simulink model "modello_calcolo_trim_1"  (R2020b)
settings: Solver=ode4  StartTime=0.0  StopTime=0.01  FixedStep=0.01  RelTol=1e-3
values from neighbouring files (symbols this model uses):
  alphavec_rad = deg2rad(alphavec)    [v2021_10_27_calcoloAerodinamica.m]
  b = 2.62    [AENEA2.m]    (also in v2021_10_27_calcoloAerodinamica.m)
  betavec_rad = deg2rad(betavec)    [v2021_10_27_calcoloAerodinamica.m]
  c = .32    (= 0.32)    [AENEA2.m]    (also in calcoloPolari.m = dim(2); v2021_10_27_calcoloAerodinamica.m)
  cbar = .32    (= 0.32)    [v2021_10_27_calcoloAerodinamica.m]
  CD0 = 0.024    [v2021_10_27_calcoloAerodinamica.m]
  CldA = KCldA(1)*180/pi    [AENEA2.m]
  CLdE = KCLdE(1)*180/pi    [AENEA2.m]
  CldR = KCldR(1)*180/pi    [AENEA2.m]
  Clp = -0.4318    [v2021_10_27_calcoloAerodinamica.m]
  CLq = 8.13    [v2021_10_27_calcoloAerodinamica.m]
  Clr = 0.1459    [v2021_10_27_calcoloAerodinamica.m]
  CmdE = KCmdE(1)*180/pi    [AENEA2.m]
  Cmq = -23.24    [v2021_10_27_calcoloAerodinamica.m]
  CndA = KCndA(1)*180/pi    [AENEA2.m]
  CndR = KCndR(1)*180/pi    [AENEA2.m]
  Cnp = 0.007507    [v2021_10_27_calcoloAerodinamica.m]
  Cnr = -0.4872    [v2021_10_27_calcoloAerodinamica.m]
  CYp = 0.050728    [v2021_10_27_calcoloAerodinamica.m]
  CYr = 0.358925    [v2021_10_27_calcoloAerodinamica.m]
  deltaAtrim = 0    [v2021_10_27_avvioSITL.m]
  deltaEtrim = 0    [v2021_10_27_avvioSITL.m]
  deltaRtrim = 0    [v2021_10_27_avvioSITL.m]
  deltaTtrim = 0.1    [v2021_10_27_avvioSITL.m]
  Dprop = 2*Rprop    (= 0.5334)    [v2021_10_27_calcoloAerodinamica.m]
  Jeng = 0    [v2021_10_27_calcoloAerodinamica.m]
  Jprop = mprop*(Dprop^2)/12    (= 0.00422031414)    [v2021_10_27_calcoloAerodinamica.m]
  rACtG = rACtP-rGP    [v2021_10_27_calcoloAerodinamica.m]
  rACwG = rACwP-rGP    [v2021_10_27_calcoloAerodinamica.m]
  rAHRSG = rAHRSP-rGP    [v2021_10_27_calcoloAerodinamica.m]
  rho = P/(287.05*T)    (= 1.16123787958)    [AENEA2.m]    (also in modello_appr_long.m = 1.164; v2021_10_27_calcoloAerodinamica.m = 1.2133)
  rLEG = rLEP-rGP    [v2021_10_27_calcoloAerodinamica.m]
  rmglG = rmglP-rGP    [v2021_10_27_calcoloAerodinamica.m]
  rmgrG = rmgrP-rGP    [v2021_10_27_calcoloAerodinamica.m]
  rngG = rngP-rGP    [v2021_10_27_calcoloAerodinamica.m]
  rNPG = rNPP-rGP    [v2021_10_27_calcoloAerodinamica.m]
  rPG = -rGP    [v2021_10_27_calcoloAerodinamica.m]
  Rprop = 0.2667    [v2021_10_27_calcoloAerodinamica.m]
  S = b*c    (= 0.8384)    [AENEA2.m]    (also in v2021_10_27_calcoloAerodinamica.m)
  W = m*g    [v2021_10_27_calcoloAerodinamica.m]
  Zeng = rPG(3)    [v2021_10_27_calcoloAerodinamica.m]
undefined symbols (not defined in the file or in its folder): CYdA, CYdR, matricepolinomi
libraries: shared6dof x1, aerolibasang x1, simulink x1
settings Model: Creator=Giorgio  LastModifiedBy=39334
settings DataIOCC: ReturnWorkspaceOutputs=off
settings OptimizationCC: BlockReduction=off  OptimizeBlockIOStorage=off  BufferReuse=off  GlobalBufferReuse=off  ExpressionFolding=off  LocalBlockOutputs=off  OptimizeDataStoreBuffers=off  BusAssignmentInplaceUpdate=off
settings DebuggingCC: InitInArrayFormatMsg=none  ArithmeticOperatorsInVariantConditions=warning
settings SFSimCC: CustomCodeUndefinedFunction=UseInterfaceOnly

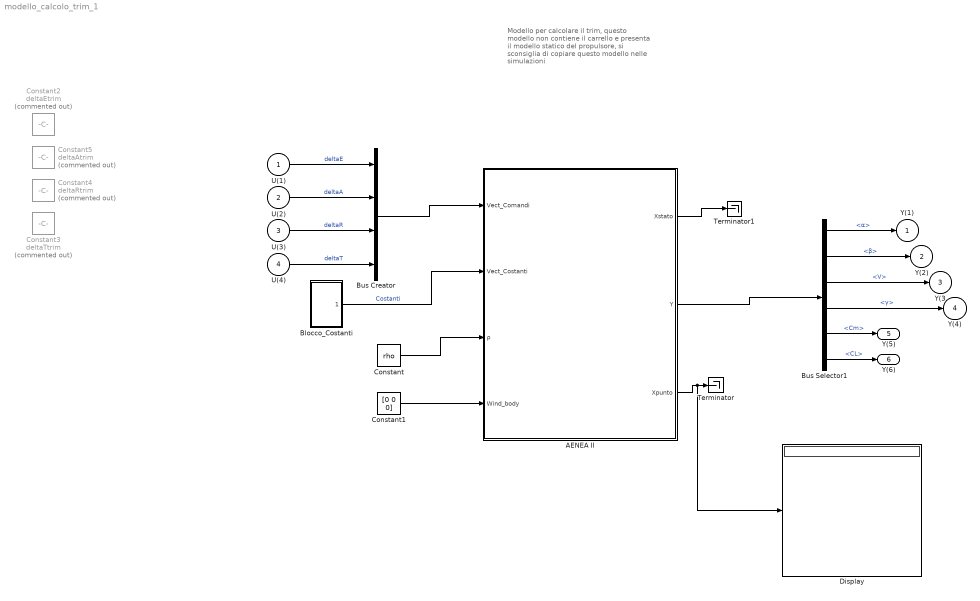
== system modello_calcolo_trim_1 ==
  note: Modello per calcolare il trim, questo modello non contiene il carrello e presenta il modello statico del propulsore, si sconsiglia di copiare questo modello nelle simulazioni
  U(1) : Inport
  U(2) : Inport  Port=2
  U(3) : Inport  Port=3
  U(4) : Inport  Port=4
  "AENEA II " : Subsystem
  Blocco_Costanti : Subsystem
  Bus Creator : BusCreator  Inputs=4
  Bus Selector1 : BusSelector  OutputSignals=Vbpolare.α,Vbpolare.β,Vbpolare.V,γ,Cm,CL
  Constant : Constant  Value=rho
  Constant1 : Constant  Value=[0 0 0]
  Constant2 : Constant  Commented=on  Value=deltaEtrim
  Constant3 : Constant  Commented=on  Value=deltaTtrim
  Constant4 : Constant  Commented=on  Value=deltaRtrim
  Constant5 : Constant  Commented=on  Value=deltaAtrim
  Display : Display
  Terminator : Terminator
  Terminator1 : Terminator
  Y(1) : Outport  VectorParamsAs1DForOutWhenUnconnected=off
  Y(2) : Outport  Port=2  VectorParamsAs1DForOutWhenUnconnected=off
  Y(3 : Outport  Port=3  VectorParamsAs1DForOutWhenUnconnected=off
  Y(4) : Outport  Port=4  VectorParamsAs1DForOutWhenUnconnected=off
  Y(5) : Outport  Port=5  VectorParamsAs1DForOutWhenUnconnected=off
  Y(6) : Outport  Port=6  VectorParamsAs1DForOutWhenUnconnected=off
  wires:
  Blocco_Costanti/1(Vect_Costanti) -> "AENEA II "/2(Vect_Costanti)  "Costanti"
  Constant/1 -> "AENEA II "/3(ρ)
  Bus Creator/1 -> "AENEA II "/1(Vect_Comandi)
  U(2)/1 -> Bus Creator/2  "deltaA"
  U(3)/1 -> Bus Creator/3  "deltaR"
  U(4)/1 -> Bus Creator/4  "deltaT"
  U(1)/1 -> Bus Creator/1  "deltaE"
  "AENEA II "/2(Y) -> Bus Selector1/1
  Bus Selector1/1 -> Y(1)/1  "<α>"
  Bus Selector1/2 -> Y(2)/1  "<β>"
  Bus Selector1/3 -> Y(3/1  "<V>"
  Bus Selector1/4 -> Y(4)/1  "<γ>"
  "AENEA II "/1(Xstato) -> Terminator1/1
  Constant1/1 -> "AENEA II "/4(Wind_body)
  "AENEA II "/3(Xpunto) -> Display/1, Terminator/1
  Bus Selector1/5 -> Y(5)/1  "<Cm>"
  Bus Selector1/6 -> Y(6)/1  "<CL>"

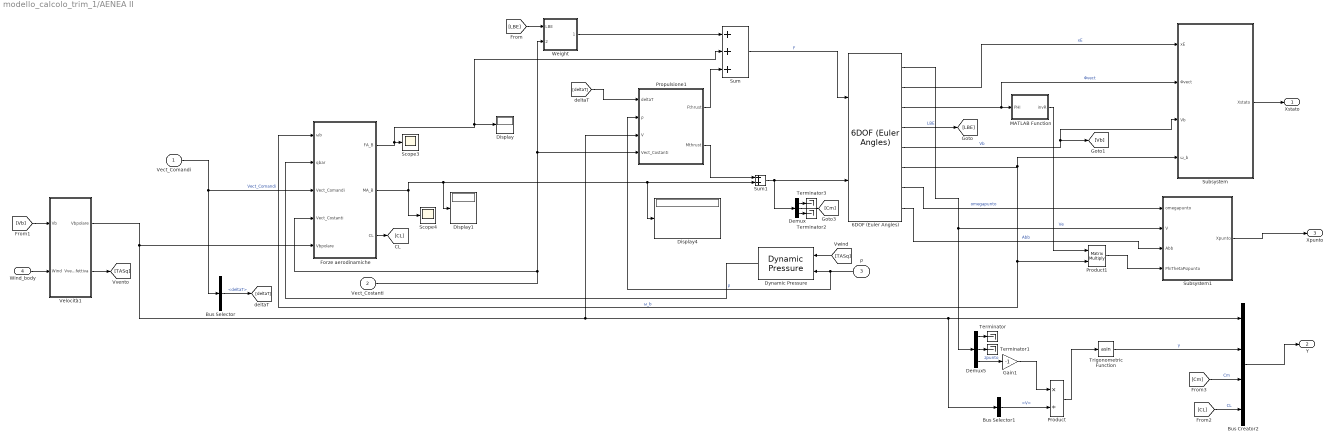
== system modello_calcolo_trim_1/AENEA II  ==
  Vect_Comandi : Inport
  Vect_Costanti : Inport  Port=2
  ρ : Inport  Port=3
  Wind_body : Inport  Port=4
  6DOF (Euler Angles) : shared6dof/6DOF (Euler Angles)  units=Metric (MKS)  mtype=Fixed  rep=Euler Angles  xme_0=State0.Pos0  Vm_0=State0.Vb0  eul_0=State0.PHI0  pm_0=State0.Omega0  mass_0=m  mass_e=0.5  mass_f=2.0  inertia=I  inertia_e=eye(3)  inertia_f=2*eye(3)  k_quat=1.0  vre_flag=on  abi_flag=off  aMode=aMode  xme_statename=''  Vm_statename=''  eul_statename=''  quat_statename=''  pm_statename=''  mass_statename=''
      settings: SourceProductBaseCode=AE,PW,MT,UV,VE,VP
  Bus Creator2 : BusCreator  Inputs=4
  Bus Selector : BusSelector  OutputSignals=deltaT
  Bus Selector1 : BusSelector  OutputSignals=V
  Demux : Demux  Outputs=3
  Demux5 : Demux  Outputs=3
  Display : Display
  Display1 : Display
  Display4 : Display
  Dynamic Pressure : aerolibasang/Dynamic Pressure
  Forze aerodinamiche : Subsystem
  Gain1 : Gain  Gain=-1
  MATLAB Function : MATLAB Function  TreatAsAtomicUnit=on
  Product : Product  Inputs=*/
  Product1 : Product  Multiplication=Matrix(*)
  Propulsione1 : Subsystem
  Scope3 : Scope
  Scope4 : Scope
  Subsystem : Subsystem
  Subsystem1 : Subsystem
  Sum : Sum  Inputs=+++
  Sum1 : Sum  Inputs=2
  Terminator{,1..3} (4 alike) : Terminator
  Trigonometric Function : Trigonometry  Operator=asin
  Velocità1 : Subsystem
  Weight : Subsystem
  Xstato : Outport  VectorParamsAs1DForOutWhenUnconnected=off
  Y : Outport  Port=2  VectorParamsAs1DForOutWhenUnconnected=off
  Xpunto : Outport  Port=3  VectorParamsAs1DForOutWhenUnconnected=off
  wires:
  Sum/1 -> 6DOF (Euler Angles)/1  "F"
  6DOF (Euler Angles)/5 -> Subsystem/3(Vb), [Vb]  "Vb"
  6DOF (Euler Angles)/6 -> Forze aerodinamiche/1(ωb), Product1/2, Subsystem/4(ω_b)  "ω_b"
  6DOF (Euler Angles)/4 -> [LBE]  "LBE"
  Forze aerodinamiche/1(FA_B) -> Sum/2, Display/1, Scope3/1
  Forze aerodinamiche/2(MA_B) -> Display4/1, Sum1/2, Display1/1, Scope4/1
  6DOF (Euler Angles)/1 -> Demux5/1, Subsystem1/2(V)  "Ve"
  Dynamic Pressure/1 -> Forze aerodinamiche/2(qbar)
  Sum1/1 -> 6DOF (Euler Angles)/2, Demux/1
  Weight/1("Forzapeso ") -> Sum/1
  [LBE] -> Weight/1(LBE)
  Vect_Comandi/1 -> Bus Selector/1, Forze aerodinamiche/3(Vect_Comandi)  "Vect_Comandi"
  Bus Selector/1 -> [deltaT]  "<deltaT>"
  Bus Creator2/1 -> Y/1
  Gain1/1 -> Product/1
  Product/1 -> Trigonometric Function/1
  Trigonometric Function/1 -> Bus Creator2/2  "γ"
  ρ/1 -> Propulsione1/2(ρ), Dynamic Pressure/2  "ρ"
  Velocità1/1(Vbpolare) -> Propulsione1/3(V), Bus Selector1/1, Bus Creator2/1, Forze aerodinamiche/5("Vbpolare ")
  [Vb] -> Velocità1/1(Vb)
  6DOF (Euler Angles)/3 -> Subsystem/2(Φvect), MATLAB Function/1(PHI)  "Φvect"
  Bus Selector1/1 -> Product/2  "<V>"
  Wind_body/1 -> Velocità1/2(Wind)
  Forze aerodinamiche/3(CL) -> [CL]
  [Cm] -> Bus Creator2/3  "Cm"
  [CL] -> Bus Creator2/4  "CL"
  6DOF (Euler Angles)/2 -> Subsystem/1(xE)  "xE"
  Subsystem/1("Xstato ") -> Xstato/1
  Demux5/2 -> Terminator1/1
  Demux5/1 -> Terminator/1
  Demux5/3 -> Gain1/1  "zpunto"
  6DOF (Euler Angles)/7 -> Subsystem1/1(omegapunto)  "omegapunto"
  6DOF (Euler Angles)/8 -> Subsystem1/3(Abb)  "Abb"
  Subsystem1/1(Xpunto) -> Xpunto/1
  Product1/1 -> Subsystem1/4("PhiThetaPsipunto ")
  MATLAB Function/1(invR) -> Product1/1
  [deltaT] -> Propulsione1/1("deltaT ")
  Vect_Costanti/1 -> Forze aerodinamiche/4(Vect_Costanti), Weight/2(Vect_Costanti), Propulsione1/4(Vect_Costanti)
  Propulsione1/2(Mthrust) -> Sum1/1
  Propulsione1/1("Fthrust ") -> Sum/3
  Demux/2 -> [Cm]
  Demux/3 -> Terminator2/1
  Demux/1 -> Terminator3/1
  Velocità1/2("Vvento_effettiva ") -> [TASq]
  [TASq] -> Dynamic Pressure/1

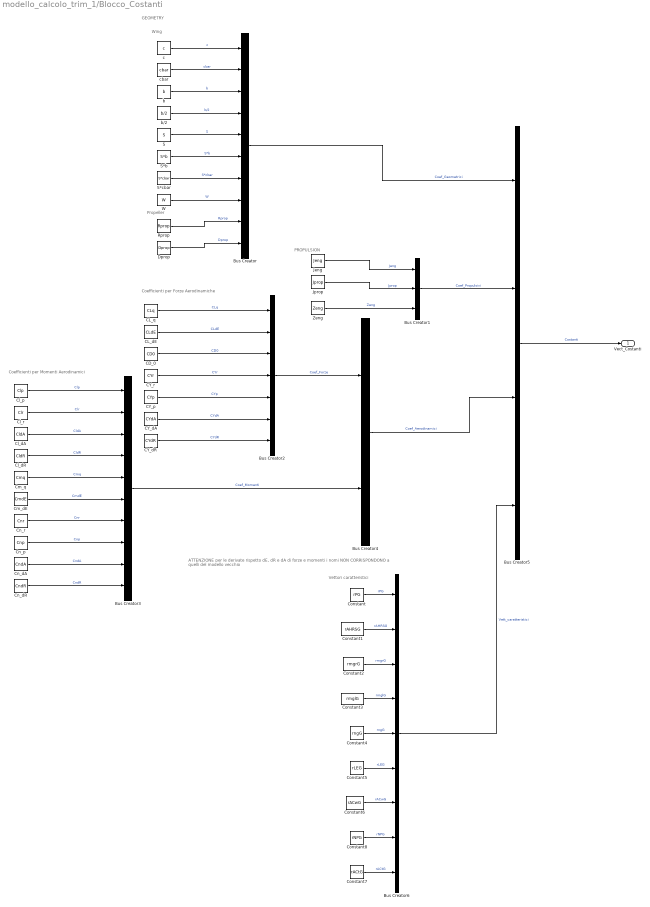
== system modello_calcolo_trim_1/Blocco_Costanti ==
  note: Vettori caratteristici
  note: ATTENZIONE per le derivate rispetto dE, dR e dA di forze e momenti i nomi NON CORRISPONDONO a quelli del modello vecchio
  note: Coefficienti per Forze Aerodinamiche
  note: Coefficienti per Momenti Aerodinamici
  note: Wing
  note: Propeller
  note: PROPULSION
  note: GEOMETRY
  Bus Creator : BusCreator  Inputs=10
  Bus Creator1 : BusCreator  Inputs=3
  Bus Creator2 : BusCreator  Inputs=7
  Bus Creator3 : BusCreator  Inputs=10
  Bus Creator4 : BusCreator  Inputs=2
  Bus Creator5 : BusCreator  Inputs=4
  Bus Creator6 : BusCreator  Inputs=9
  CD_0 : Constant  Value=CD0
  "CL_dE " : Constant  Value=CLdE
  "CL_q " : Constant  Value=CLq
  CY_dA : Constant  Value=CYdA
  CY_dR : Constant  Value=CYdR
  "CY_p " : Constant  Value=CYp
  CY_r : Constant  Value=CYr
  Cl_dA : Constant  Value=CldA
  Cl_dR : Constant  Value=CldR
  "Cl_p " : Constant  Value=Clp
  "Cl_r " : Constant  Value=Clr
  "Cm_dE " : Constant  Value=CmdE
  "Cm_q " : Constant  Value=Cmq
  Cn_dA : Constant  Value=CndA
  "Cn_dR " : Constant  Value=CndR
  "Cn_p " : Constant  Value=Cnp
  "Cn_r " : Constant  Value=Cnr
  Constant : Constant  Value=rPG
  Constant1 : Constant  Value=rAHRSG
  Constant2 : Constant  Value=rmgrG
  Constant3 : Constant  Value=rmglG
  Constant4 : Constant  Value=rngG
  Constant5 : Constant  Value=rLEG
  Constant6 : Constant  Value=rACwG
  Constant7 : Constant  Value=rACtG
  Constant8 : Constant  Value=rNPG
  Dprop : Constant  Value=Dprop
  Jeng : Constant  Value=Jeng
  Jprop : Constant  Value=Jprop
  Rprop : Constant  Value=Rprop
  S : Constant  Value=S
  "S*b " : Constant  Value=S*b
  S*cbar : Constant  Value=S*cbar
  W : Constant  Value=W
  Zeng : Constant  Value=Zeng
  b : Constant  Value=b
  b/2 : Constant  Value=b/2
  c : Constant  Value=c
  "cbar " : Constant  Value=cbar
  Vect_Costanti : Outport  VectorParamsAs1DForOutWhenUnconnected=off
  wires:
  "CY_p "/1 -> Bus Creator2/5  "CYp"
  Cl_dR/1 -> Bus Creator3/4  "CldR"
  "Cn_dR "/1 -> Bus Creator3/10  "CndR"
  "CL_q "/1 -> Bus Creator2/1  "CLq"
  "Cn_p "/1 -> Bus Creator3/8  "Cnp"
  Bus Creator1/1 -> Bus Creator5/2  "Coef_Propulsivi"
  CD_0/1 -> Bus Creator2/3  "CD0"
  Bus Creator4/1 -> Bus Creator5/3  "Coef_Aerodinamici"
  "Cm_dE "/1 -> Bus Creator3/6  "CmdE"
  "Cn_r "/1 -> Bus Creator3/7  "Cnr"
  "Cl_r "/1 -> Bus Creator3/2  "Clr"
  "Cm_q "/1 -> Bus Creator3/5  "Cmq"
  CY_dR/1 -> Bus Creator2/7  "CYdR"
  Cl_dA/1 -> Bus Creator3/3  "CldA"
  CY_dA/1 -> Bus Creator2/6  "CYdA"
  "CL_dE "/1 -> Bus Creator2/2  "CLdE"
  Dprop/1 -> Bus Creator/10  "Dprop"
  Cn_dA/1 -> Bus Creator3/9  "CndA"
  Bus Creator5/1 -> Vect_Costanti/1  "Costanti"
  Bus Creator/1 -> Bus Creator5/1  "Coef_Geometrici"
  Jeng/1 -> Bus Creator1/1  "Jeng"
  c/1 -> Bus Creator/1  "c"
  "S*b "/1 -> Bus Creator/6  "S*b"
  W/1 -> Bus Creator/8  "W"
  Rprop/1 -> Bus Creator/9  "Rprop"
  b/1 -> Bus Creator/3  "b"
  Bus Creator3/1 -> Bus Creator4/2  "Coef_Momenti"
  Bus Creator2/1 -> Bus Creator4/1  "Coef_Forze"
  S*cbar/1 -> Bus Creator/7  "S*cbar"
  Jprop/1 -> Bus Creator1/2  "Jprop"
  b/2/1 -> Bus Creator/4  "b/2"
  "Cl_p "/1 -> Bus Creator3/1  "Clp"
  CY_r/1 -> Bus Creator2/4  "CYr"
  S/1 -> Bus Creator/5  "S"
  "cbar "/1 -> Bus Creator/2  "cbar"
  Zeng/1 -> Bus Creator1/3  "Zeng"
  Constant/1 -> Bus Creator6/1  "rPG"
  Bus Creator6/1 -> Bus Creator5/4  "Vett_caratteristici"
  Constant3/1 -> Bus Creator6/4  "rmglG"
  Constant8/1 -> Bus Creator6/8  "rNPG"
  Constant6/1 -> Bus Creator6/7  "rACwG"
  Constant5/1 -> Bus Creator6/6  "rLEG"
  Constant4/1 -> Bus Creator6/5  "rngG"
  Constant7/1 -> Bus Creator6/9  "rACtG"
  Constant2/1 -> Bus Creator6/3  "rmgrG"
  Constant1/1 -> Bus Creator6/2  "rAHRSG"

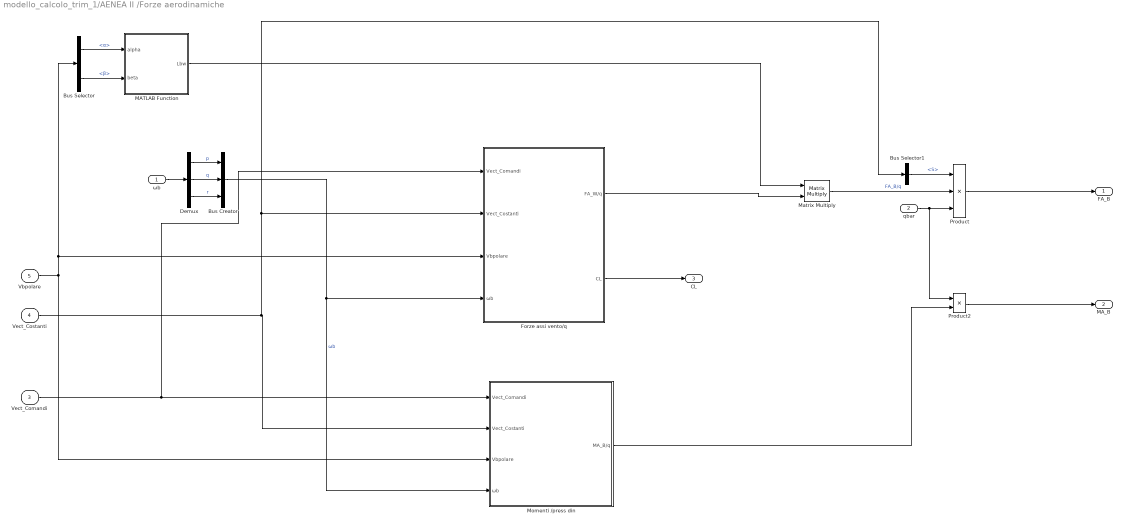
== system modello_calcolo_trim_1/AENEA II /Forze aerodinamiche ==
  ωb : Inport
  qbar : Inport  Port=2
  Vect_Comandi : Inport  Port=3
  Vect_Costanti : Inport  Port=4
  "Vbpolare " : Inport  Port=5
  Bus Creator : BusCreator  Inputs=3
  Bus Selector : BusSelector  OutputSignals=α,β
  Bus Selector1 : BusSelector  OutputSignals=Coef_Geometrici.S
  Demux : Demux  Outputs=3
  Forze assi vento/q : Subsystem
  MATLAB Function : MATLAB Function  TreatAsAtomicUnit=on
  Matrix Multiply : Product  Multiplication=Matrix(*)
  Momenti /press din : Subsystem
  Product : Product  Inputs=3
  Product2 : Product
  FA_B : Outport  VectorParamsAs1DForOutWhenUnconnected=off
  MA_B : Outport  Port=2  VectorParamsAs1DForOutWhenUnconnected=off
  CL : Outport  Port=3  VectorParamsAs1DForOutWhenUnconnected=off
  wires:
  Product2/1 -> MA_B/1
  Product/1 -> FA_B/1
  qbar/1 -> Product/3, Product2/1
  ωb/1 -> Demux/1
  Demux/1 -> Bus Creator/1  "p"
  Demux/2 -> Bus Creator/2  "q"
  Demux/3 -> Bus Creator/3  "r"
  Bus Selector/1 -> MATLAB Function/1(alpha)  "<α>"
  Bus Selector/2 -> MATLAB Function/2(beta)  "<β>"
  MATLAB Function/1(Lbw) -> Matrix Multiply/1
  Matrix Multiply/1 -> Product/2  "FA_B/q"
  Momenti /press din/1(MA_B/q) -> Product2/2
  Forze assi vento/q/1(FA_W/q) -> Matrix Multiply/2
  Vect_Comandi/1 -> Forze assi vento/q/1(Vect_Comandi), Momenti /press din/1(Vect_Comandi)
  "Vbpolare "/1 -> Bus Selector/1, Forze assi vento/q/3("Vbpolare "), Momenti /press din/3("Vbpolare ")
  Bus Creator/1 -> Momenti /press din/4(ωb), Forze assi vento/q/4(ωb)  "ωb"
  Vect_Costanti/1 -> Bus Selector1/1, Forze assi vento/q/2(Vect_Costanti), Momenti /press din/2(Vect_Costanti)
  Bus Selector1/1 -> Product/1  "<S>"
  Forze assi vento/q/2(CL) -> CL/1

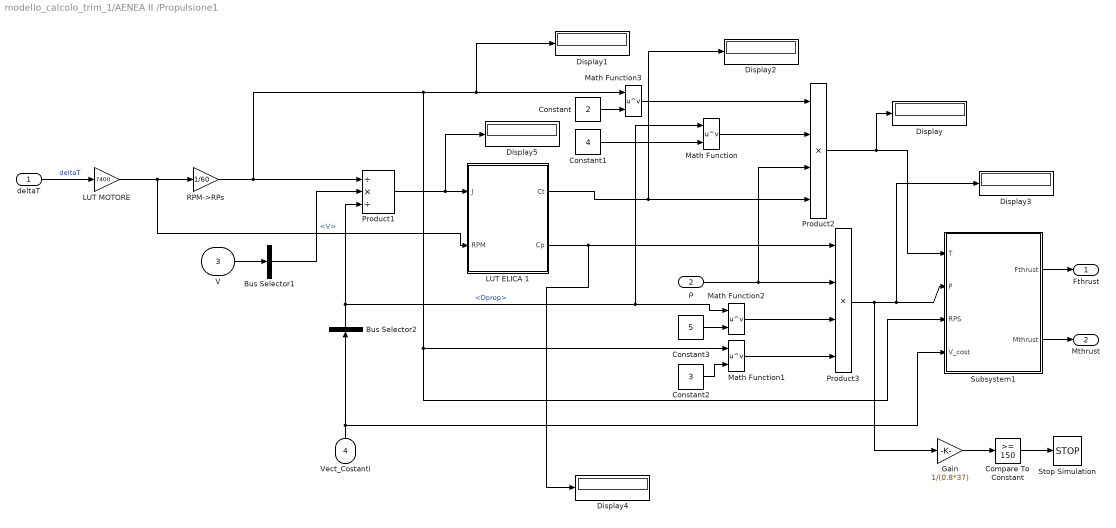
== system modello_calcolo_trim_1/AENEA II /Propulsione1 ==
  "deltaT " : Inport
  ρ : Inport  Port=2
  V : Inport  Port=3
  Vect_Costanti : Inport  Port=4
  Bus Selector1 : BusSelector  OutputSignals=V
  Bus Selector2 : BusSelector  OutputSignals=Coef_Geometrici.Dprop
  Compare To Constant : simulink/Logic and Bit Operations/Compare To Constant  relop=>=  const=150  OutDataTypeStr=boolean
  Constant : Constant  Value=2
  Constant1 : Constant  Value=4
  Constant2 : Constant  Value=3
  Constant3 : Constant  Value=5
  Display{,1..5} (6 alike) : Display
  Gain : Gain  Gain=1/(0.8*37)
  LUT ELICA 1 : Subsystem
  LUT MOTORE : Gain  Gain=7400
  Math Function{,1..3} (4 alike) : Math  Operator=pow  SignedPower=on  SaturateOnIntegerOverflow=on
  Product1 : Product  Inputs=/*/
  Product2 : Product  Inputs=****
  Product3 : Product  Inputs=****
  RPM->RPs : Gain  Gain=1/60
  Stop Simulation : Stop
  Subsystem1 : Subsystem
  "Fthrust " : Outport  VectorParamsAs1DForOutWhenUnconnected=off
  Mthrust : Outport  Port=2  VectorParamsAs1DForOutWhenUnconnected=off
  wires:
  Vect_Costanti/1 -> Subsystem1/4(V_cost), Bus Selector2/1
  "deltaT "/1 -> LUT MOTORE/1  "deltaT"
  LUT MOTORE/1 -> LUT ELICA 1/2(RPM), RPM->RPs/1
  V/1 -> Bus Selector1/1
  Bus Selector1/1 -> Product1/2  "<V>"
  RPM->RPs/1 -> Subsystem1/3(RPS), Math Function1/1, Display1/1, Math Function3/1, Product1/1
  Bus Selector2/1 -> Math Function2/1, Math Function/1, Product1/3  "<Dprop>"
  Product1/1 -> LUT ELICA 1/1(J), Display5/1
  ρ/1 -> Product2/3, Product3/2
  LUT ELICA 1/2(Cp) -> Display4/1, Product3/1
  LUT ELICA 1/1(Ct) -> Display2/1, Product2/4
  Math Function3/1 -> Product2/1
  Math Function/1 -> Product2/2
  Constant/1 -> Math Function3/2
  Constant1/1 -> Math Function/2
  Math Function2/1 -> Product3/3
  Constant3/1 -> Math Function2/2
  Constant2/1 -> Math Function1/2
  Math Function1/1 -> Product3/4
  Product2/1 -> Display/1, Subsystem1/1(T)
  Subsystem1/1(Fthrust) -> "Fthrust "/1
  Subsystem1/2("Mthrust ") -> Mthrust/1
  Product3/1 -> Gain/1, Display3/1, Subsystem1/2(P)
  Gain/1 -> Compare To Constant/1
  Compare To Constant/1 -> Stop Simulation/1

== system modello_calcolo_trim_1/AENEA II /Subsystem ==
  xE : Inport
  Φvect : Inport  Port=2
  Vb : Inport  Port=3
  ω_b : Inport  Port=4
  Bus Creator1 : BusCreator  Inputs=4
  Bus Creator{3..4,8..9} (4 alike) : BusCreator  Inputs=3
  Demux{1..2,6..7} (4 alike) : Demux  Outputs=3
  "Xstato " : Outport  VectorParamsAs1DForOutWhenUnconnected=off
  wires:
  Demux2/3 -> Bus Creator4/3  "r"
  Bus Creator4/1 -> Bus Creator1/3  "ωvect"
  Φvect/1 -> Demux6/1
  Vb/1 -> Demux7/1
  Bus Creator8/1 -> Bus Creator1/2  "PhiThetaPsi"
  Demux1/3 -> Bus Creator3/3  "h"
  Demux2/2 -> Bus Creator4/2  "q"
  Demux2/1 -> Bus Creator4/1  "p"
  Bus Creator3/1 -> Bus Creator1/4  "xyz"
  ω_b/1 -> Demux2/1
  Demux6/3 -> Bus Creator8/3  "Psi"
  Demux6/1 -> Bus Creator8/1  "Phi"
  Demux1/1 -> Bus Creator3/1  "x"
  Demux7/1 -> Bus Creator9/1  "u"
  Demux7/3 -> Bus Creator9/3  "w"
  Bus Creator9/1 -> Bus Creator1/1  "uvw"
  Demux1/2 -> Bus Creator3/2  "y"
  Demux7/2 -> Bus Creator9/2  "v"
  Demux6/2 -> Bus Creator8/2  "Theta"
  Bus Creator1/1 -> "Xstato "/1  "Xstato"
  xE/1 -> Demux1/1

== system modello_calcolo_trim_1/AENEA II /Subsystem1 ==
  omegapunto : Inport
  V : Inport  Port=2
  Abb : Inport  Port=3
  "PhiThetaPsipunto " : Inport  Port=4
  Bus Creator{5,7,10..11} (4 alike) : BusCreator  Inputs=3
  Bus Creator6 : BusCreator  Inputs=4
  Demux{3..4,8..9} (4 alike) : Demux  Outputs=3
  Xpunto : Outport  VectorParamsAs1DForOutWhenUnconnected=off
  wires:
  Demux4/3 -> Bus Creator7/3  "wpunto"
  Demux3/1 -> Bus Creator5/1  "ppunto"
  Demux4/2 -> Bus Creator7/2  "vpunto"
  Demux8/2 -> Bus Creator10/2  "Thetapunto"
  Bus Creator10/1 -> Bus Creator6/2  "EulerAnglespunto"
  Demux3/2 -> Bus Creator5/2  "qpunto"
  Demux4/1 -> Bus Creator7/1  "upunto"
  V/1 -> Demux9/1
  Demux8/1 -> Bus Creator10/1  "Phipunto"
  Bus Creator11/1 -> Bus Creator6/4  "xyzpunto"
  Demux8/3 -> Bus Creator10/3  "Psipunto"
  Demux3/3 -> Bus Creator5/3  "rpunto"
  Demux9/2 -> Bus Creator11/2  "Yepunto"
  Bus Creator7/1 -> Bus Creator6/1  "Vbpunto"
  Bus Creator5/1 -> Bus Creator6/3  "ωpunto"
  Demux9/1 -> Bus Creator11/1  "Xepunto"
  Demux9/3 -> Bus Creator11/3  "Zepunto"
  "PhiThetaPsipunto "/1 -> Demux8/1
  omegapunto/1 -> Demux3/1
  Abb/1 -> Demux4/1
  Bus Creator6/1 -> Xpunto/1

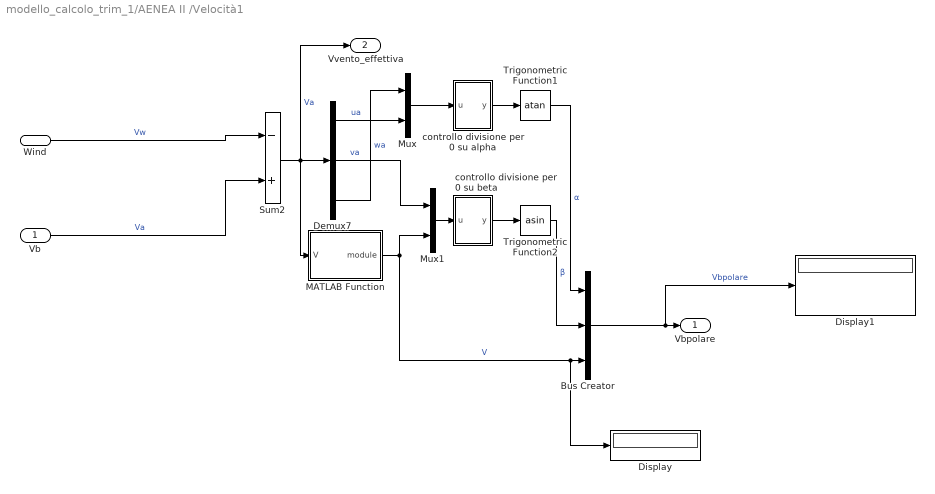
== system modello_calcolo_trim_1/AENEA II /Velocità1 ==
  Vb : Inport
  Wind : Inport  Port=2
  Bus Creator : BusCreator  Inputs=3
  Demux7 : Demux  Outputs=3
  Display : Display
  Display1 : Display
  MATLAB Function : MATLAB Function  TreatAsAtomicUnit=on
  Mux : Mux  Inputs=2
  Mux1 : Mux  Inputs=2
  Sum2 : Sum  Inputs=-+
  Trigonometric Function1 : Trigonometry  Operator=atan
  Trigonometric Function2 : Trigonometry  Operator=asin
  controllo divisione per 0 su alpha : MATLAB Function  TreatAsAtomicUnit=on
  controllo divisione per 0 su beta : MATLAB Function  TreatAsAtomicUnit=on
  Vbpolare : Outport  VectorParamsAs1DForOutWhenUnconnected=off
  "Vvento_effettiva " : Outport  Port=2  VectorParamsAs1DForOutWhenUnconnected=off
  wires:
  Bus Creator/1 -> Display1/1, Vbpolare/1  "Vbpolare"
  Trigonometric Function1/1 -> Bus Creator/1  "α"
  MATLAB Function/1(module) -> Mux1/2, Display/1, Bus Creator/3  "V"
  controllo divisione per 0 su alpha/1(y) -> Trigonometric Function1/1
  controllo divisione per 0 su beta/1(y) -> Trigonometric Function2/1
  Trigonometric Function2/1 -> Bus Creator/2  "β"
  Vb/1 -> Sum2/2  "Va"
  Sum2/1 -> "Vvento_effettiva "/1, MATLAB Function/1(V), Demux7/1  "Va"
  Mux/1 -> controllo divisione per 0 su alpha/1(u)
  Demux7/3 -> Mux/1  "wa"
  Demux7/1 -> Mux/2  "ua"
  Mux1/1 -> controllo divisione per 0 su beta/1(u)
  Demux7/2 -> Mux1/1  "va"
  Wind/1 -> Sum2/1  "Vw"

== system modello_calcolo_trim_1/AENEA II /Weight ==
  LBE : Inport
  Vect_Costanti : Inport  Port=2
  Bus Selector : BusSelector  OutputSignals=Coef_Geometrici.W
  Display3 : Display
  Product3 : Product  Multiplication=Matrix(*)
  "Forzapeso " : Outport  VectorParamsAs1DForOutWhenUnconnected=off
  wires:
  Product3/1 -> "Forzapeso "/1, Display3/1
  LBE/1 -> Product3/1
  Vect_Costanti/1 -> Bus Selector/1
  Bus Selector/1 -> Product3/2  "<W>"

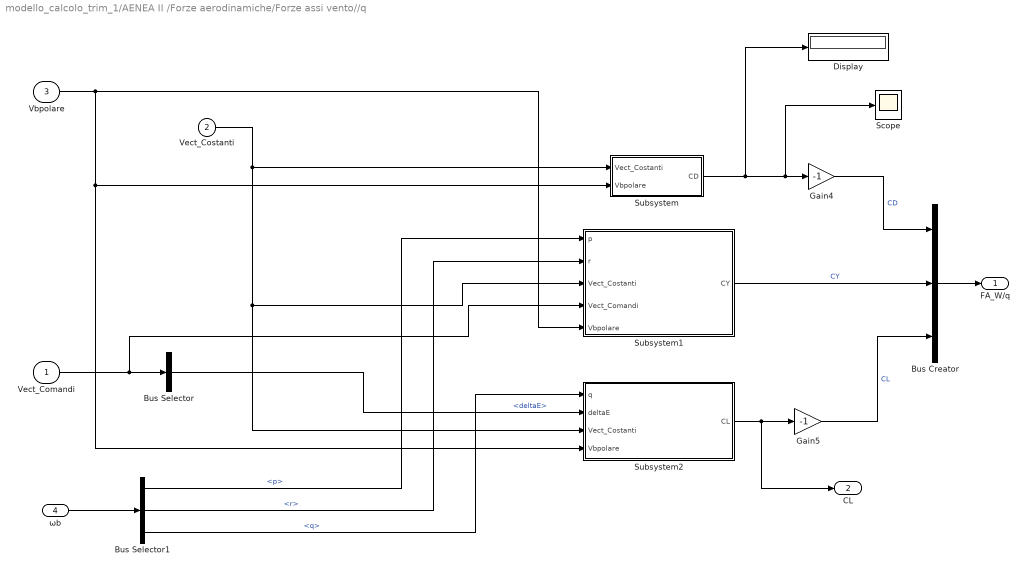
== system modello_calcolo_trim_1/AENEA II /Forze aerodinamiche/Forze assi vento//q ==
  Vect_Comandi : Inport
  Vect_Costanti : Inport  Port=2
  "Vbpolare " : Inport  Port=3
  ωb : Inport  Port=4
  Bus Creator : BusCreator  Inputs=3
  Bus Selector : BusSelector  OutputSignals=deltaE
  Bus Selector1 : BusSelector  OutputSignals=p,r,q
  Display : Display
  Gain4 : Gain  Gain=-1
  Gain5 : Gain  Gain=-1
  Scope : Scope
  Subsystem : Subsystem
  Subsystem1 : Subsystem
  Subsystem2 : Subsystem
  FA_W/q : Outport  VectorParamsAs1DForOutWhenUnconnected=off
  CL : Outport  Port=2  VectorParamsAs1DForOutWhenUnconnected=off
  wires:
  Bus Selector/1 -> Subsystem2/2(deltaE)  "<deltaE>"
  Subsystem/1(CD) -> Display/1, Scope/1, Gain4/1
  Subsystem2/1(CL) -> CL/1, Gain5/1
  Vect_Costanti/1 -> Subsystem2/3(Vect_Costanti), Subsystem1/3(Vect_Costanti), Subsystem/1(Vect_Costanti)
  Vect_Comandi/1 -> Subsystem1/4(Vect_Comandi), Bus Selector/1
  "Vbpolare "/1 -> Subsystem1/5("Vbpolare "), Subsystem2/4("Vbpolare "), Subsystem/2("Vbpolare ")
  ωb/1 -> Bus Selector1/1
  Bus Selector1/1 -> Subsystem1/1(p)  "<p>"
  Bus Selector1/3 -> Subsystem2/1(q)  "<q>"
  Bus Selector1/2 -> Subsystem1/2(r)  "<r>"
  Bus Creator/1 -> FA_W/q/1
  Gain5/1 -> Bus Creator/3  "CL"
  Subsystem1/1("CY ") -> Bus Creator/2  "CY"
  Gain4/1 -> Bus Creator/1  "CD"

== system modello_calcolo_trim_1/AENEA II /Forze aerodinamiche/Momenti //press din ==
  Vect_Comandi : Inport
  Vect_Costanti : Inport  Port=2
  "Vbpolare " : Inport  Port=3
  ωb : Inport  Port=4
  Bus Creator : BusCreator  Inputs=3
  Bus Selector : BusSelector  OutputSignals=Coef_Geometrici.S*b,Coef_Geometrici.S*cbar
  Product : Product
  Product1 : Product
  Product3 : Product
  Subsystem3 : Subsystem
  Subsystem4 : Subsystem
  Subsystem5 : Subsystem
  MA_B/q : Outport  VectorParamsAs1DForOutWhenUnconnected=off
  wires:
  Subsystem5/1(Cn) -> Product3/2
  Subsystem4/1(Cm) -> Product1/2
  Subsystem3/1(Cl) -> Product/2
  Vect_Costanti/1 -> Bus Selector/1, Subsystem3/1(Vect_Costanti), Subsystem5/1(Vect_Costanti), Subsystem4/1(Vect_Costanti)
  Vect_Comandi/1 -> Subsystem4/2(Vect_Comandi), Subsystem3/2(Vect_Comandi), Subsystem5/2(Vect_Comandi)
  "Vbpolare "/1 -> Subsystem5/3("Vbpolare "), Subsystem4/3("Vbpolare "), Subsystem3/3("Vbpolare ")
  ωb/1 -> Subsystem5/4(ωb), Subsystem4/4(ωb), Subsystem3/4(ωb)
  Bus Selector/1 -> Product3/1, Product/1  "<S*b>"
  Bus Selector/2 -> Product1/1  "<S*cbar>"
  Bus Creator/1 -> MA_B/q/1
  Product/1 -> Bus Creator/1  "Cl"
  Product1/1 -> Bus Creator/2  "Cm"
  Product3/1 -> Bus Creator/3  "Cn"

== system modello_calcolo_trim_1/AENEA II /Propulsione1/LUT ELICA 1 ==
  J : Inport
  RPM : Inport  Port=2
  Constant : Constant  Value=matricepolinomi  VectorParams1D=off
  MATLAB Function : MATLAB Function  TreatAsAtomicUnit=on
  Ct : Outport  VectorParamsAs1DForOutWhenUnconnected=off
  Cp : Outport  Port=2  VectorParamsAs1DForOutWhenUnconnected=off
  wires:
  MATLAB Function/2(Cp) -> Cp/1  "Cp"
  J/1 -> MATLAB Function/1(J)
  Constant/1 -> MATLAB Function/3(matricepolinomi)
  MATLAB Function/1(Ct) -> Ct/1  "Ct"
  RPM/1 -> MATLAB Function/2(RPM)

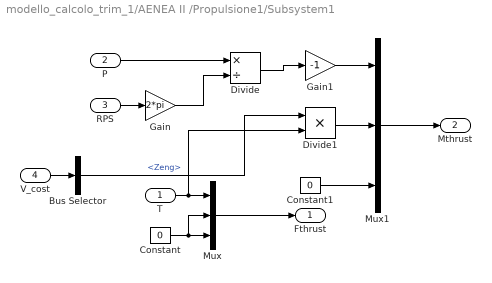
== system modello_calcolo_trim_1/AENEA II /Propulsione1/Subsystem1 ==
  T : Inport
  P : Inport  Port=2
  RPS : Inport  Port=3
  V_cost : Inport  Port=4
  Bus Selector : BusSelector  OutputSignals=Coef_Propulsivi.Zeng
  Constant : Constant  Value=0
  Constant1 : Constant  Value=0
  Divide : Product  Inputs=*/
  Divide1 : Product  Inputs=**
  Gain : Gain  Gain=2*pi
  Gain1 : Gain  Gain=-1
  Mux : Mux  Inputs=3
  Mux1 : Mux  Inputs=3
  Fthrust : Outport  VectorParamsAs1DForOutWhenUnconnected=off
  "Mthrust " : Outport  Port=2  VectorParamsAs1DForOutWhenUnconnected=off
  wires:
  T/1 -> Divide1/2, Mux/1
  Constant/1 -> Mux/2, Mux/3
  Mux/1 -> Fthrust/1
  RPS/1 -> Gain/1
  P/1 -> Divide/1
  Gain/1 -> Divide/2
  Gain1/1 -> Mux1/1
  Divide/1 -> Gain1/1
  Divide1/1 -> Mux1/2
  Constant1/1 -> Mux1/3
  Mux1/1 -> "Mthrust "/1
  V_cost/1 -> Bus Selector/1
  Bus Selector/1 -> Divide1/1  "<Zeng>"

== system modello_calcolo_trim_1/AENEA II /Forze aerodinamiche/Forze assi vento//q/Subsystem ==
  note: CD=CD(alpha_x,beta)
  Vect_Costanti : Inport
  "Vbpolare " : Inport  Port=2
  2-D Lookup Table : Lookup_n-D  BreakpointsForDimension1=alphavec_rad  BreakpointsForDimension2=betavec_rad  Table=CD(2:end,2:end)  InternalRulePriority=Speed  RndMeth=Simplest  InputSameDT=on
      settings: InputPortMap=u0,u1
  Bus Selector : BusSelector  OutputSignals=Coef_Aerodinamici.Coef_Forze.CD0
  Bus Selector1 : BusSelector  OutputSignals=α,β
  Sum1 : Sum  Inputs=|++
  CD : Outport  VectorParamsAs1DForOutWhenUnconnected=off
  wires:
  2-D Lookup Table/1 -> Sum1/1
  Sum1/1 -> CD/1
  Bus Selector/1 -> Sum1/2  "<CD0>"
  Vect_Costanti/1 -> Bus Selector/1
  Bus Selector1/1 -> 2-D Lookup Table/1  "<α>"
  "Vbpolare "/1 -> Bus Selector1/1
  Bus Selector1/2 -> 2-D Lookup Table/2  "<β>"

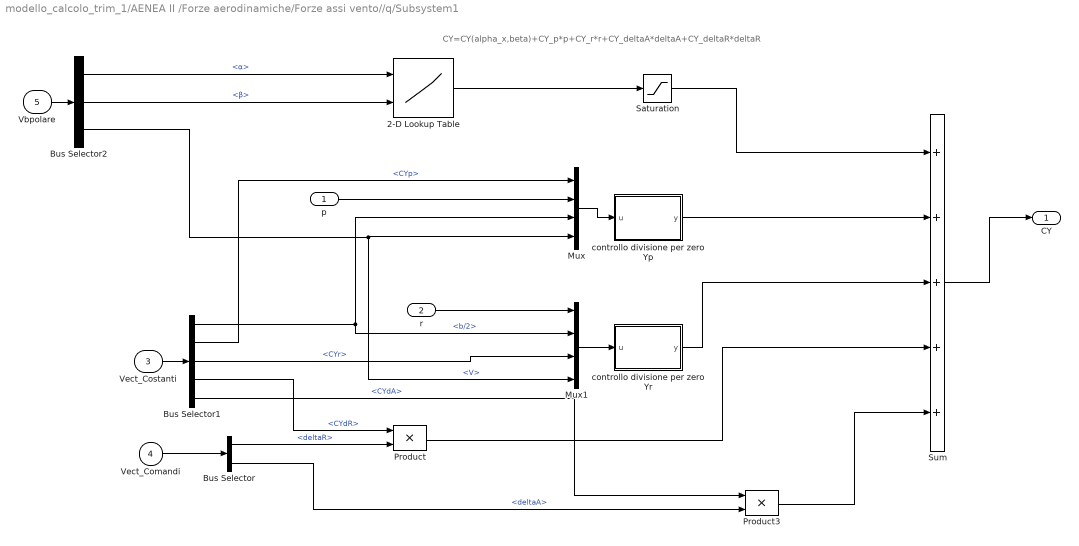
== system modello_calcolo_trim_1/AENEA II /Forze aerodinamiche/Forze assi vento//q/Subsystem1 ==
  note: CY=CY(alpha_x,beta)+CY_p*p+CY_r*r+CY_deltaA*deltaA+CY_deltaR*deltaR
  p : Inport
  r : Inport  Port=2
  Vect_Costanti : Inport  Port=3
  Vect_Comandi : Inport  Port=4
  "Vbpolare " : Inport  Port=5
  2-D Lookup Table : Lookup_n-D  BreakpointsForDimension1=alphavec_rad  BreakpointsForDimension2=betavec_rad  Table=CY(2:end,2:end)  InternalRulePriority=Speed  RndMeth=Simplest  InputSameDT=on
      settings: InputPortMap=u0,u1
  Bus Selector : BusSelector  OutputSignals=deltaR,deltaA
  Bus Selector1 : BusSelector  OutputSignals=Coef_Geometrici.b/2,Coef_Aerodinamici.Coef_Forze.CYp,Coef_Aerodinamici.Coef_Forze.CYr,Coef_Aerodinamici.Coef_Forze.CYdR,Coef_Aerodinamici.Coef_Forze.CYdA
  Bus Selector2 : BusSelector  OutputSignals=α,β,V
  Mux : Mux
  Mux1 : Mux
  Product : Product
  Product3 : Product
  Saturation : Saturate  UpperLimit=0.1  LowerLimit=-0.1
  Sum : Sum  Inputs=5
  "controllo divisione per zero Yp " : MATLAB Function  TreatAsAtomicUnit=on
  controllo divisione per zero Yr : MATLAB Function  TreatAsAtomicUnit=on
  "CY " : Outport  VectorParamsAs1DForOutWhenUnconnected=off
  wires:
  Bus Selector1/2 -> Mux/1  "<CYp>"
  p/1 -> Mux/2
  "controllo divisione per zero Yp "/1(y) -> Sum/2
  Sum/1 -> "CY "/1
  r/1 -> Mux1/1
  2-D Lookup Table/1 -> Saturation/1
  Bus Selector1/4 -> Product/1  "<CYdR>"
  Bus Selector/1 -> Product/2  "<deltaR>"
  Bus Selector1/5 -> Product3/1  "<CYdA>"
  Bus Selector/2 -> Product3/2  "<deltaA>"
  Product/1 -> Sum/4
  Product3/1 -> Sum/5
  Vect_Comandi/1 -> Bus Selector/1
  Vect_Costanti/1 -> Bus Selector1/1
  Bus Selector1/3 -> Mux1/3  "<CYr>"
  Bus Selector1/1 -> Mux/3, Mux1/2  "<b/2>"
  Bus Selector2/1 -> 2-D Lookup Table/1  "<α>"
  "Vbpolare "/1 -> Bus Selector2/1
  Bus Selector2/3 -> Mux/4, Mux1/4  "<V>"
  Bus Selector2/2 -> 2-D Lookup Table/2  "<β>"
  Mux/1 -> "controllo divisione per zero Yp "/1(u)
  Mux1/1 -> controllo divisione per zero Yr/1(u)
  controllo divisione per zero Yr/1(y) -> Sum/3
  Saturation/1 -> Sum/1

== system modello_calcolo_trim_1/AENEA II /Forze aerodinamiche/Forze assi vento//q/Subsystem2 ==
  note: CL=CL(ALPHA_X,BETA)+CL_q*q+CL_de*de
  q : Inport
  deltaE : Inport  Port=2
  Vect_Costanti : Inport  Port=3
  "Vbpolare " : Inport  Port=4
  2-D Lookup Table : Lookup_n-D  BreakpointsForDimension1=alphavec_rad  BreakpointsForDimension2=betavec_rad  Table=CL(2:end,2:end)  InternalRulePriority=Speed  RndMeth=Simplest  InputSameDT=on
      settings: InputPortMap=u0,u1
  Bus Selector : BusSelector  OutputSignals=Coef_Aerodinamici.Coef_Forze.CLq,Coef_Aerodinamici.Coef_Forze.CLdE,Coef_Geometrici.cbar
  Bus Selector1 : BusSelector  OutputSignals=α,β,V
  Gain1 : Gain  Gain=2
  Mux : Mux
  Product4 : Product
  Sum : Sum  Inputs=3
  "controllo divisione per zero Lq " : MATLAB Function  TreatAsAtomicUnit=on
  CL : Outport  VectorParamsAs1DForOutWhenUnconnected=off
  wires:
  Sum/1 -> CL/1
  q/1 -> Mux/2
  Bus Selector/1 -> Mux/1  "<CLq>"
  Bus Selector/2 -> Product4/1  "<CLdE>"
  deltaE/1 -> Product4/2
  "controllo divisione per zero Lq "/1(y) -> Sum/2
  Product4/1 -> Sum/3
  2-D Lookup Table/1 -> Sum/1
  Vect_Costanti/1 -> Bus Selector/1
  Gain1/1 -> Mux/4
  Bus Selector/3 -> Mux/3  "<cbar>"
  Bus Selector1/1 -> 2-D Lookup Table/1  "<α>"
  "Vbpolare "/1 -> Bus Selector1/1
  Bus Selector1/3 -> Gain1/1  "<V>"
  Bus Selector1/2 -> 2-D Lookup Table/2  "<β>"
  Mux/1 -> "controllo divisione per zero Lq "/1(u)

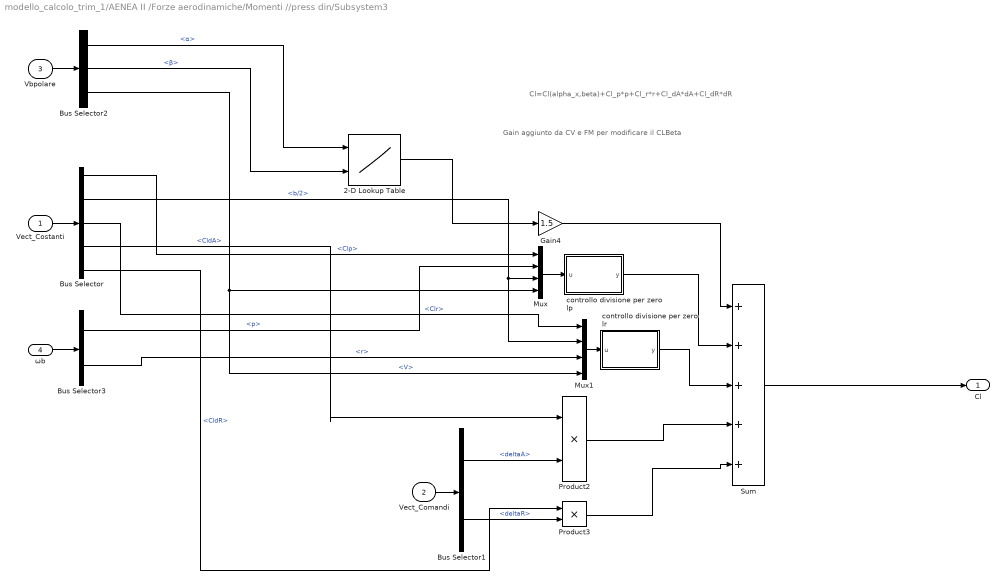
== system modello_calcolo_trim_1/AENEA II /Forze aerodinamiche/Momenti //press din/Subsystem3 ==
  note: Gain aggiunto da CV e FM per modificare il CLBeta
  note: Cl=Cl(alpha_x,beta)+Cl_p*p+Cl_r*r+Cl_dA*dA+Cl_dR*dR
  Vect_Costanti : Inport
  Vect_Comandi : Inport  Port=2
  "Vbpolare " : Inport  Port=3
  ωb : Inport  Port=4
  2-D Lookup Table : Lookup_n-D  BreakpointsForDimension1=alphavec_rad  BreakpointsForDimension2=betavec_rad  Table=Cl(2:end,2:end)  InternalRulePriority=Speed  RndMeth=Simplest  InputSameDT=on
      settings: InputPortMap=u0,u1
  Bus Selector : BusSelector  OutputSignals=Coef_Aerodinamici.Coef_Momenti.Clp,Coef_Geometrici.b/2,Coef_Aerodinamici.Coef_Momenti.Clr,Coef_Aerodinamici.Coef_Momenti.CldA,Coef_Aerodinamici.Coef_Momenti.CldR
  Bus Selector1 : BusSelector  OutputSignals=deltaA,deltaR
  Bus Selector2 : BusSelector  OutputSignals=α,β,V
  Bus Selector3 : BusSelector  OutputSignals=p,r
  Gain4 : Gain  Gain=1.5
  Mux : Mux
  Mux1 : Mux
  Product2 : Product
  Product3 : Product
  Sum : Sum  Inputs=5
  "controllo divisione per zero lp " : MATLAB Function  TreatAsAtomicUnit=on
  "controllo divisione per zero lr " : MATLAB Function  TreatAsAtomicUnit=on
  Cl : Outport  VectorParamsAs1DForOutWhenUnconnected=off
  wires:
  Sum/1 -> Cl/1
  Bus Selector/3 -> Mux1/1  "<Clr>"
  Bus Selector1/2 -> Product3/2  "<deltaR>"
  Bus Selector1/1 -> Product2/2  "<deltaA>"
  Product3/1 -> Sum/5
  Product2/1 -> Sum/4
  "controllo divisione per zero lp "/1(y) -> Sum/2
  2-D Lookup Table/1 -> Gain4/1
  Gain4/1 -> Sum/1
  Vect_Costanti/1 -> Bus Selector/1
  Bus Selector/1 -> Mux/1  "<Clp>"
  Bus Selector/5 -> Product3/1  "<CldR>"
  Bus Selector/4 -> Product2/1  "<CldA>"
  Bus Selector/2 -> Mux1/2, Mux/3  "<b/2>"
  Vect_Comandi/1 -> Bus Selector1/1
  Bus Selector2/1 -> 2-D Lookup Table/1  "<α>"
  "Vbpolare "/1 -> Bus Selector2/1
  Bus Selector2/3 -> Mux1/4, Mux/4  "<V>"
  Bus Selector2/2 -> 2-D Lookup Table/2  "<β>"
  ωb/1 -> Bus Selector3/1
  Bus Selector3/1 -> Mux/2  "<p>"
  Bus Selector3/2 -> Mux1/3  "<r>"
  Mux/1 -> "controllo divisione per zero lp "/1(u)
  Mux1/1 -> "controllo divisione per zero lr "/1(u)
  "controllo divisione per zero lr "/1(y) -> Sum/3

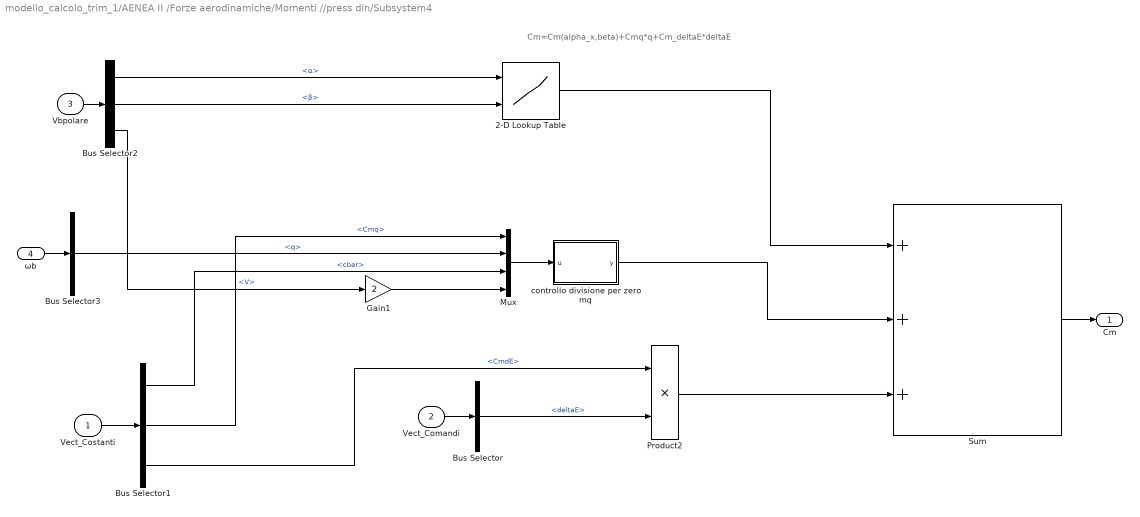
== system modello_calcolo_trim_1/AENEA II /Forze aerodinamiche/Momenti //press din/Subsystem4 ==
  note: Cm=Cm(alpha_x,beta)+Cmq*q+Cm_deltaE*deltaE
  Vect_Costanti : Inport
  Vect_Comandi : Inport  Port=2
  "Vbpolare " : Inport  Port=3
  ωb : Inport  Port=4
  2-D Lookup Table : Lookup_n-D  BreakpointsForDimension1=alphavec_rad  BreakpointsForDimension2=betavec_rad  Table=Cm(2:end,2:end)  InternalRulePriority=Speed  RndMeth=Simplest  InputSameDT=on
      settings: InputPortMap=u0,u1
  Bus Selector : BusSelector  OutputSignals=deltaE
  Bus Selector1 : BusSelector  OutputSignals=Coef_Geometrici.cbar,Coef_Aerodinamici.Coef_Momenti.Cmq,Coef_Aerodinamici.Coef_Momenti.CmdE
  Bus Selector2 : BusSelector  OutputSignals=α,β,V
  Bus Selector3 : BusSelector  OutputSignals=q
  Gain1 : Gain  Gain=2
  Mux : Mux
  Product2 : Product
  Sum : Sum  Inputs=3
  "controllo divisione per zero mq " : MATLAB Function  TreatAsAtomicUnit=on
  Cm : Outport  VectorParamsAs1DForOutWhenUnconnected=off
  wires:
  Bus Selector1/2 -> Mux/1  "<Cmq>"
  Sum/1 -> Cm/1
  Gain1/1 -> Mux/4
  Bus Selector1/3 -> Product2/1  "<CmdE>"
  Bus Selector/1 -> Product2/2  "<deltaE>"
  Product2/1 -> Sum/3
  2-D Lookup Table/1 -> Sum/1
  Vect_Comandi/1 -> Bus Selector/1
  Vect_Costanti/1 -> Bus Selector1/1
  Bus Selector1/1 -> Mux/3  "<cbar>"
  Bus Selector2/3 -> Gain1/1  "<V>"
  "Vbpolare "/1 -> Bus Selector2/1
  Bus Selector2/1 -> 2-D Lookup Table/1  "<α>"
  Bus Selector2/2 -> 2-D Lookup Table/2  "<β>"
  ωb/1 -> Bus Selector3/1
  Bus Selector3/1 -> Mux/2  "<q>"
  Mux/1 -> "controllo divisione per zero mq "/1(u)
  "controllo divisione per zero mq "/1(y) -> Sum/2

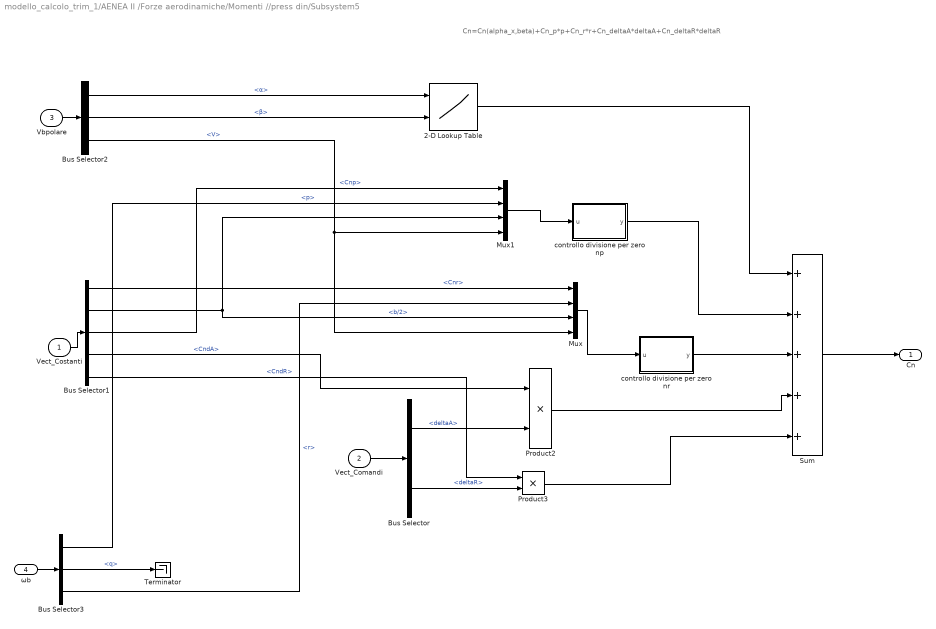
== system modello_calcolo_trim_1/AENEA II /Forze aerodinamiche/Momenti //press din/Subsystem5 ==
  note: Cn=Cn(alpha_x,beta)+Cn_p*p+Cn_r*r+Cn_deltaA*deltaA+Cn_deltaR*deltaR
  Vect_Costanti : Inport
  Vect_Comandi : Inport  Port=2
  "Vbpolare " : Inport  Port=3
  ωb : Inport  Port=4
  2-D Lookup Table : Lookup_n-D  BreakpointsForDimension1=alphavec_rad  BreakpointsForDimension2=betavec_rad  Table=Cn(2:end,2:end)  InternalRulePriority=Speed  RndMeth=Simplest  InputSameDT=on
      settings: InputPortMap=u0,u1
  Bus Selector : BusSelector  OutputSignals=deltaA,deltaR
  Bus Selector1 : BusSelector  OutputSignals=Coef_Aerodinamici.Coef_Momenti.Cnr,Coef_Geometrici.b/2,Coef_Aerodinamici.Coef_Momenti.Cnp,Coef_Aerodinamici.Coef_Momenti.CndA,Coef_Aerodinamici.Coef_Momenti.CndR
  Bus Selector2 : BusSelector  OutputSignals=α,β,V
  Bus Selector3 : BusSelector  OutputSignals=p,q,r
  Mux : Mux
  Mux1 : Mux
  Product2 : Product
  Product3 : Product
  Sum : Sum  Inputs=5
  Terminator : Terminator
  "controllo divisione per zero np " : MATLAB Function  TreatAsAtomicUnit=on
  "controllo divisione per zero nr " : MATLAB Function  TreatAsAtomicUnit=on
  Cn : Outport  VectorParamsAs1DForOutWhenUnconnected=off
  wires:
  Bus Selector1/3 -> Mux1/1  "<Cnp>"
  Product2/1 -> Sum/4
  Product3/1 -> Sum/5
  Sum/1 -> Cn/1
  Bus Selector1/1 -> Mux/1  "<Cnr>"
  Bus Selector1/5 -> Product3/1  "<CndR>"
  Bus Selector/2 -> Product3/2  "<deltaR>"
  Bus Selector/1 -> Product2/2  "<deltaA>"
  2-D Lookup Table/1 -> Sum/1
  Vect_Comandi/1 -> Bus Selector/1
  Vect_Costanti/1 -> Bus Selector1/1
  Bus Selector1/4 -> Product2/1  "<CndA>"
  Bus Selector1/2 -> Mux1/3, Mux/3  "<b/2>"
  Bus Selector2/3 -> Mux1/4, Mux/4  "<V>"
  "Vbpolare "/1 -> Bus Selector2/1
  Bus Selector2/1 -> 2-D Lookup Table/1  "<α>"
  Bus Selector2/2 -> 2-D Lookup Table/2  "<β>"
  ωb/1 -> Bus Selector3/1
  Bus Selector3/3 -> Mux/2  "<r>"
  Bus Selector3/1 -> Mux1/2  "<p>"
  Bus Selector3/2 -> Terminator/1  "<q>"
  Mux/1 -> "controllo divisione per zero nr "/1(u)
  "controllo divisione per zero nr "/1(y) -> Sum/3
  Mux1/1 -> "controllo divisione per zero np "/1(u)
  "controllo divisione per zero np "/1(y) -> Sum/2

== matlab function modello_calcolo_trim_1/AENEA II /Velocità1/controllo divisione per 0 su beta ==
  data: u input; y output
function y = sinbeta(u)

if length(u)~=2
    error('vettore ingresso errato')
else
    if u(2)==0
        y=0;
    else 
        y=u(1)/u(2);
    end
end

== matlab function modello_calcolo_trim_1/AENEA II /Propulsione1/LUT ELICA 1/MATLAB Function ==
  data: J input; Ct output; RPM input; Cp output; matricepolinomi input
function [Ct,Cp] = calcolo_Ct_Cp(J,RPM,matricepolinomi)

lct00 = matricepolinomi(1,1);
lct10 = matricepolinomi(1,2);
lct01 = matricepolinomi(1,3);
lct20 = matricepolinomi(1,4);
lct11 = matricepolinomi(1,5);
lct02 = matricepolinomi(1,6);
lct30 = matricepolinomi(1,7);
lct21 = matricepolinomi(1,8);
lct12 = matricepolinomi(1,9);
lct40 = matricepolinomi(1,10);
lct31 = matricepolinomi(1,11);
lct22 = matricepolinomi(1,12);

qct00 = matricepolinomi(2,1);
qct10 = matricepolinomi(2,2);
qct01 = matricepolinomi(2,3);
qct20 = matricepolinomi(2,4);
qct11 = matricepolinomi(2,5);
qct02 = matricepolinomi(2,6);
qct30 = matricepolinomi(2,7);
qct21 = matricepolinomi(2,8);
qct12 = matricepolinomi(2,9);
qct03 = matricepolinomi(2,10);
qct40 = matricepolinomi(2,11);
qct31 = matricepolinomi(2,12);
qct22 = matricepolinomi(2,13);
qct13 = matricepolinomi(2,14);
qct04 = matricepolinomi(2,15);
qct50 = matricepolinomi(2,16);
qct41 = matricepolinomi(2,17);
qct32 = matricepolinomi(2,18);
qct23 = matricepolinomi(2,19);
qct14 = matricepolinomi(2,20);
qct05 = matricepolinomi(2,21);

cp100 = matricepolinomi(3,1);
cp110 = matricepolinomi(3,2);
cp101 = matricepolinomi(3,3);
cp120 = matricepolinomi(3,4);
cp111 = matricepolinomi(3,5);
cp102 = matricepolinomi(3,6);
cp130 = matricepolinomi(3,7);
cp121 = matricepolinomi(3,8);
cp112 = matricepolinomi(3,9);
cp140 = matricepolinomi(3,10);
cp131 = matricepolinomi(3,11);
cp122 = matricepolinomi(3,12);

cp200 = matricepolinomi(4,1);
cp210 = matricepolinomi(4,2);
cp201 = matricepolinomi(4,3);
cp220 = matricepolinomi(4,4);
cp211 = matricepolinomi(4,5);
cp202 = matricepolinomi(4,6);
cp230 = matricepolinomi(4,7);
cp221 = matricepolinomi(4,8);
cp212 = matricepolinomi(4,9);
cp240 = matricepolinomi(4,10);
cp231 = matricepolinomi(4,11);
cp222 = matricepolinomi(4,12);

cp300 = matricepolinomi(5,1);
cp310 = matricepolinomi(5,2);
cp301 = matricepolinomi(5,3);
cp320 = matricepolinomi(5,4);
cp311 = matricepolinomi(5,5);
cp302 = matricepolinomi(5,6);
cp330 = matricepolinomi(5,7);
cp321 = matricepolinomi(5,8);
cp312 = matricepolinomi(5,9);
cp340 = matricepolinomi(5,10);
cp331 = matricepolinomi(5,11);
cp322 = matricepolinomi(5,12);

cp400 = matricepolinomi(6,1);
cp410 = matricepolinomi(6,2);
cp401 = matricepolinomi(6,3);
cp420 = matricepolinomi(6,4);
cp411 = matricepolinomi(6,5);
cp402 = matricepolinomi(6,6);
cp430 = matricepolinomi(6,7);
cp421 = matricepolinomi(6,8);
cp412 = matricepolinomi(6,9);
cp440 = matricepolinomi(6,10);
cp431 = matricepolinomi(6,11);
cp422 = matricepolinomi(6,12);


if J<=0.32
    x = RPM;
    y = J;
    Ct = qct00 + qct10*x + qct01*y + qct20*x^2 + qct11*x*y + qct02*y^2 + qct30*x^3 + qct21*x^2*y + qct12*x*y^2 + qct03*y^3 + qct40*x^4 + qct31*x^3*y + qct22*x^2*y^2 + qct13*x*y^3 + qct04*y^4 + qct50*x^5 + qct41*x^4*y + qct32*x^3*y^2 + qct23*x^2*y^3 + qct14*x*y^4 + qct05*y^5;
elseif J>0.32
    x = RPM;
    y = J;
    Ct = lct00 + lct10*x + lct01*y + lct20*x^2 + lct11*x*y + lct02*y^2 + lct30*x^3 + lct21*x^2*y + lct12*x*y^2 + lct40*x^4 + lct31*x^3*y + lct22*x^2*y^2;
else
    Ct = 0;
end

if (J<=0.34)&&(RPM<=5000)
    x = RPM;
    y = J;
    Cp = cp100 + cp110*x + cp101*y + cp120*x^2 + cp111*x*y + cp102*y^2 + cp130*x^3 + cp121*x^2*y + cp112*x*y^2 + cp140*x^4 + cp131*x^3*y + cp122*x^2*y^2;
elseif (J<=0.34)&&(RPM>5000)
    x = RPM;
    y = J;
    Cp = cp200 + cp210*x + cp201*y + cp220*x^2 + cp211*x*y + cp202*y^2 + cp230*x^3 + cp221*x^2*y + cp212*x*y^2 + cp240*x^4 + cp231*x^3*y + cp222*x^2*y^2;
elseif (J>0.34)&&(RPM<=5000)
    x = RPM;
    y = J;
    Cp = cp300 + cp310*x + cp301*y + cp320*x^2 + cp311*x*y + cp302*y^2 + cp330*x^3 + cp321*x^2*y + cp312*x*y^2 + cp340*x^4 + cp331*x^3*y + cp322*x^2*y^2;
elseif (J>0.34)&&(RPM>5000)
    x = RPM;
    y = J;
    Cp = cp400 + cp410*x + cp401*y + cp420*x^2 + cp411*x*y + cp402*y^2 + cp430*x^3 + cp421*x^2*y + cp412*x*y^2 + cp440*x^4 + cp431*x^3*y + cp422*x^2*y^2;
else
    Cp = 0;
end

== matlab function modello_calcolo_trim_1/AENEA II /MATLAB Function ==
  data: PHI input; invR output
function invR = omega2PHIdot(PHI)

if length(PHI)==3
    Phi=PHI(1);
    Theta=PHI(2);
    
    invR=[1, sin(Phi)*tan(Theta), cos(Phi)*tan(Theta); 0, cos(Phi), -sin(Phi); 0, sin(Phi)*sec(Theta), cos(Phi)*sec(Theta)];
else 
    error('il vettore PHI non va bene')
end

== matlab function modello_calcolo_trim_1/AENEA II /Forze aerodinamiche/MATLAB Function ==
  data: alpha input; Lbw output; beta input
function Lbw = DCMbw(alpha,beta)


Lbw=[cos(alpha)*cos(beta), -cos(alpha)*sin(beta), -sin(alpha); sin(beta), cos(beta), 0; sin(alpha)*cos(beta), -sin(alpha)*sin(beta), cos(alpha)];

== matlab function modello_calcolo_trim_1/AENEA II /Forze aerodinamiche/Forze assi vento//q/Subsystem1/controllo divisione per zero Yp  ==
  data: u input; y output
function y = Yp(u)

if length(u)~=4
    error('vettore ingresso dimensione errata')
else
    if u(4)==0
        y=0;
    else
        y=u(1)*u(2)*u(3)/u(4);
    end
end

== matlab function modello_calcolo_trim_1/AENEA II /Forze aerodinamiche/Forze assi vento//q/Subsystem1/controllo divisione per zero Yr ==
  data: u input; y output
function y = Yr(u)

if length(u)~=4
    error('vettore ingresso dimensione errata')
else
    if u(4)==0
        y=0;
    else
        y=u(1)*u(2)*u(3)/u(4);
    end
end

== matlab function modello_calcolo_trim_1/AENEA II /Forze aerodinamiche/Forze assi vento//q/Subsystem2/controllo divisione per zero Lq  ==
  data: u input; y output
function y = Lq(u)

if length(u)~=4
    error('vettore ingresso dimensione errata')
else
    if u(4)==0
        y=0;
    else
        y=u(1)*u(2)*u(3)/u(4);
    end
end

== matlab function modello_calcolo_trim_1/AENEA II /Forze aerodinamiche/Momenti //press din/Subsystem3/controllo divisione per zero lp  ==
  data: u input; y output
function y = lp(u)

if length(u)~=4
    error('vettore ingresso dimensione errata')
else
    if u(4)==0
        y=0;
    else
        y=u(1)*u(2)*u(3)/u(4);
    end
end

== matlab function modello_calcolo_trim_1/AENEA II /Forze aerodinamiche/Momenti //press din/Subsystem3/controllo divisione per zero lr  ==
  data: u input; y output
function y = lr(u)

if length(u)~=4
    error('vettore ingresso dimensione errata')
else
    if u(4)==0
        y=0;
    else
        y=u(1)*u(2)*u(3)/u(4);
    end
end

== matlab function modello_calcolo_trim_1/AENEA II /Forze aerodinamiche/Momenti //press din/Subsystem4/controllo divisione per zero mq  ==
  data: u input; y output
function y = mq(u)

if length(u)~=4
    error('vettore ingresso dimensione errata')
else
    if u(4)==0
        y=0;
    else
        y=u(1)*u(2)*u(3)/u(4);
    end
end

== matlab function modello_calcolo_trim_1/AENEA II /Forze aerodinamiche/Momenti //press din/Subsystem5/controllo divisione per zero nr  ==
  data: u input; y output
function y = nr(u)

if length(u)~=4
    error('vettore ingresso dimensione errata')
else
    if u(4)==0
        y=0;
    else
        y=u(1)*u(2)*u(3)/u(4);
    end
end

== matlab function modello_calcolo_trim_1/AENEA II /Forze aerodinamiche/Momenti //press din/Subsystem5/controllo divisione per zero np  ==
  data: u input; y output
function y = np(u)

if length(u)~=4
    error('vettore ingresso dimensione errata')
else
    if u(4)==0
        y=0;
    else
        y=u(1)*u(2)*u(3)/u(4);
    end
end

== matlab function modello_calcolo_trim_1/AENEA II /Velocità1/MATLAB Function ==
  data: V input; module output
function module = absolute(V)


if length(V)==3
   module=sqrt((V(1)^2)+(V(2)^2)+(V(3)^2));
else 
    error('dimension of input incorrect')
end

== matlab function modello_calcolo_trim_1/AENEA II /Velocità1/controllo divisione per 0 su alpha ==
  data: u input; y output
function y = tgalpha(u)

if length(u)~=2
    error('vettore ingresso errato')
else
    if u(2)==0
        y=0;
    else 
        y=u(1)/u(2);
    end
end
